simulink model "DriveCond"  (R2020a)
settings: Solver=VariableStepAuto  StartTime=0.0  StopTime=10.0  RelTol=1e-3
settings Model: Creator=Administrator  LastModifiedBy=Administrator

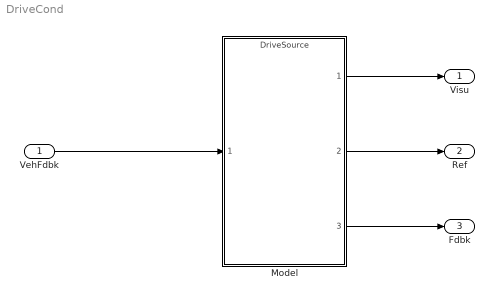
== system DriveCond ==
  VehFdbk : Inport
  Model : ModelReference  ModelNameDialog=DriveSource.slx  SimulationMode=Normal  ModelReferenceVersion=1.4
  Visu : Outport
  Ref : Outport  Port=2
  Fdbk : Outport  Port=3
  wires:
  VehFdbk/1 -> Model/1
  Model/1 -> Visu/1
  Model/2 -> Ref/1
  Model/3 -> Fdbk/1
